simulink model "codeur_qui_marche"  (R2018b)
settings: Solver=VariableStepAuto  StartTime=0.0  StopTime=3  RelTol=1e-3  EnableMultiTasking=on
values from neighbouring files (symbols this model uses):
  freq_proc = 10000    [parametres_cubli.m]
undefined symbols (not defined in the file or in its folder): K3
libraries: c2802xlib x5, c2837xDlib x4, simulink x1, c280xlib x1
settings Model: ExtModeTrigDuration=8  Creator=ntest557  LastModifiedBy=ntest557
settings OptimizationCC: DefaultUnderspecifiedDataType=single  EnhancedBackFolding=on  PassReuseOutputArgsAs=Individual arguments  MaxStackSize=512  OptimizeBlockOrder=speed  DifferentSizesBufferReuse=on  OptimizationCustomize=off
settings DebuggingCC: ParameterTunabilityLossMsg=error
settings HardwareCC: ProdBitPerChar=16  ProdBitPerInt=16  ProdBitPerPointer=32  ProdBitPerSizeT=32  ProdBitPerPtrDiffT=32  ProdLargestAtomicInteger=Integer  ProdLargestAtomicFloat=None  ProdWordSize=16  ProdLongLongMode=on  ProdHWDeviceType=Texas Instruments->C2000
settings SFSimCC: MATLABDynamicMemAlloc=off
settings RTWCC: SystemTargetFile=ert.tlc  HardwareBoard=TI Delfino F28379D LaunchPad  TemplateMakefile=ert_default_tmf  GenerateReport=on  Toolchain=Texas Instruments Code Composer Studio (C2000)  IncludeHyperlinkInReport=on  LaunchReport=on  GenerateTraceInfo=on  GenerateTraceReport=on  GenerateTraceReportSl=on  GenerateTraceReportSf=on  GenerateTraceReportEml=on
settings CodeAppCC: ForceParamTrailComments=on  IgnoreCustomStorageClasses=off  OperatorAnnotations=on  SimulinkDataObjDesc=on  SFDataObjDesc=on  InsertBlockDesc=on
settings ERTTargetCC: CodeReplacementLibrary=TI C28x

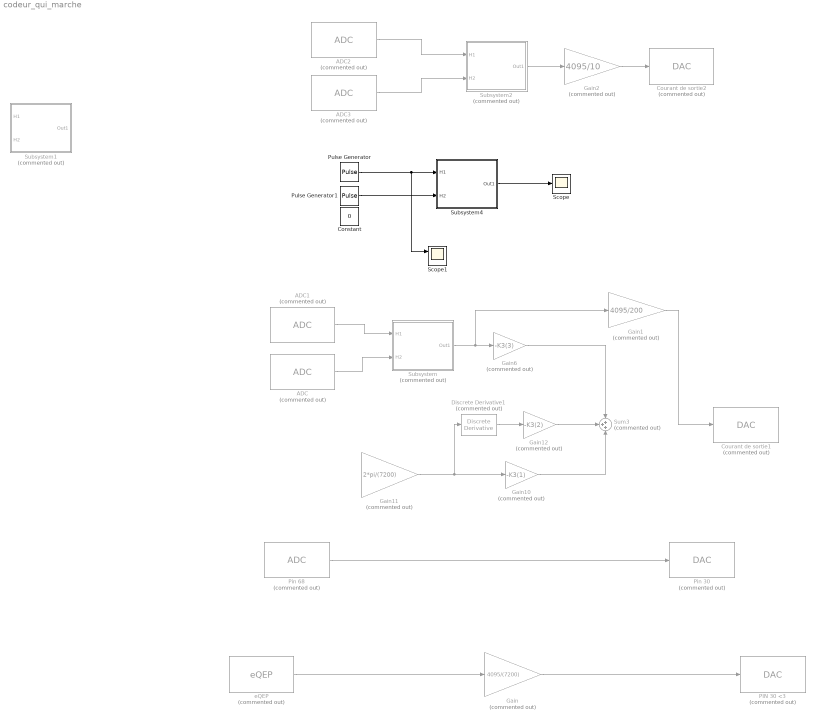
== system codeur_qui_marche ==
  ADC : c2802xlib/ADC  Commented=on  ADCModule=B  samplingMode=Single sample mode  ADCResolution=12-bit (Single-ended input)  useSOC1=SOC0  useSOC2=SOC0_SOC1  SOCAcquisitionWindow=15  SOCTriggerSource=Software  SOCInterruptTrigger=No ADCINT  Ts=1/freq_proc  dType=uint16  postInterrupt=off  interruptSel=ADCINT1  ADCINTContinuous=on  endma=off  chdma=1  blkParamProc=C2000_Type4  conv1=ADCINA0  conv2=ADCINA0 and ADCINB0  conv1_Type4=ADCIN3  conv2_Type4=ADCIN0 and ADCIN1
      settings: SourceProductName=Embedded Coder Support Package for Texas Instruments C2000 Processors
  ADC1 : c2802xlib/ADC  Commented=on  ADCModule=C  samplingMode=Single sample mode  ADCResolution=12-bit (Single-ended input)  useSOC1=SOC0  useSOC2=SOC0_SOC1  SOCAcquisitionWindow=15  SOCTriggerSource=Software  SOCInterruptTrigger=No ADCINT  Ts=1/freq_proc  dType=uint16  postInterrupt=off  interruptSel=ADCINT1  ADCINTContinuous=on  endma=off  chdma=1  blkParamProc=C2000_Type4  conv1=ADCINA0  conv2=ADCINA0 and ADCINB0  conv1_Type4=ADCIN3  conv2_Type4=ADCIN0 and ADCIN1
      settings: SourceProductName=Embedded Coder Support Package for Texas Instruments C2000 Processors
  ADC2 : c2802xlib/ADC  Commented=on  ADCModule=C  samplingMode=Single sample mode  ADCResolution=12-bit (Single-ended input)  useSOC1=SOC0  useSOC2=SOC0_SOC1  SOCAcquisitionWindow=15  SOCTriggerSource=Software  SOCInterruptTrigger=No ADCINT  Ts=1/freq_proc  dType=uint16  postInterrupt=off  interruptSel=ADCINT1  ADCINTContinuous=on  endma=off  chdma=1  blkParamProc=C2000_Type4  conv1=ADCINA0  conv2=ADCINA0 and ADCINB0  conv1_Type4=ADCIN3  conv2_Type4=ADCIN0 and ADCIN1
      settings: SourceProductName=Embedded Coder Support Package for Texas Instruments C2000 Processors
  ADC3 : c2802xlib/ADC  Commented=on  ADCModule=B  samplingMode=Single sample mode  ADCResolution=12-bit (Single-ended input)  useSOC1=SOC0  useSOC2=SOC0_SOC1  SOCAcquisitionWindow=15  SOCTriggerSource=Software  SOCInterruptTrigger=No ADCINT  Ts=1/freq_proc  dType=uint16  postInterrupt=off  interruptSel=ADCINT1  ADCINTContinuous=on  endma=off  chdma=1  blkParamProc=C2000_Type4  conv1=ADCINA0  conv2=ADCINA0 and ADCINB0  conv1_Type4=ADCIN3  conv2_Type4=ADCIN0 and ADCIN1
      settings: SourceProductName=Embedded Coder Support Package for Texas Instruments C2000 Processors
  Constant : Constant  Value=0
  Courant de sortie1 : c2837xDlib/DAC  Commented=on  channel=A  saturate=off
      settings: SourceProductName=Embedded Coder Support Package for Texas Instruments C2000 Processors  SourceProductBaseCode=TIC2000
  Courant de sortie2 : c2837xDlib/DAC  Commented=on  channel=A  saturate=off
      settings: SourceProductName=Embedded Coder Support Package for Texas Instruments C2000 Processors  SourceProductBaseCode=TIC2000
  Discrete Derivative1 : simulink/Discrete/Discrete Derivative  Commented=on  gainval=1.0  ICPrevScaledInput=0.0  OutMin=[]  OutMax=[]  OutDataType=fixdt(1, 16)  OutScaling=2^-10  DoSatur=off
  Gain : Gain  Commented=on  Gain=4095/(7200)
  Gain1 : Gain  Commented=on  Gain=4095/200
  Gain10 : Gain  Commented=on  Gain=-K3(1)
  Gain11 : Gain  Commented=on  Gain=2*pi/(7200)
  Gain12 : Gain  Commented=on  Gain=-K3(2)
  Gain2 : Gain  Commented=on  Gain=4095/10
  Gain6 : Gain  Commented=on  Gain=-K3(3)
  PIN 30 <3 : c2837xDlib/DAC  Commented=on  channel=A  saturate=off
      settings: SourceProductName=Embedded Coder Support Package for Texas Instruments C2000 Processors  SourceProductBaseCode=TIC2000
  Pin 30 : c2837xDlib/DAC  Commented=on  channel=A  saturate=off
      settings: SourceProductName=Embedded Coder Support Package for Texas Instruments C2000 Processors  SourceProductBaseCode=TIC2000
  "Pin 68 " : c2802xlib/ADC  Commented=on  ADCModule=B  samplingMode=Single sample mode  ADCResolution=12-bit (Single-ended input)  useSOC1=SOC0  useSOC2=SOC0_SOC1  SOCAcquisitionWindow=15  SOCTriggerSource=Software  SOCInterruptTrigger=No ADCINT  Ts=0.001  dType=uint16  postInterrupt=off  interruptSel=ADCINT1  ADCINTContinuous=on  endma=off  chdma=1  blkParamProc=C2000_Type4  conv1=ADCINA0  conv2=ADCINA0 and ADCINB0  conv1_Type4=ADCIN4  conv2_Type4=ADCIN0 and ADCIN1
      settings: SourceProductName=Embedded Coder Support Package for Texas Instruments C2000 Processors
  Pulse Generator : DiscretePulseGenerator  PulseType=Time based  Period=0.1  PulseWidth=50
  Pulse Generator1 : DiscretePulseGenerator  PulseType=Time based  Period=0.1  PulseWidth=50  PhaseDelay=2*0.1/3
  Scope : Scope
  Scope1 : Scope  NumInputPorts=2
  Subsystem : Subsystem  Commented=on
  Subsystem1 : Subsystem  Commented=on
  Subsystem2 : Subsystem  Commented=on
  Subsystem4 : Subsystem
  Sum3 : Sum  Commented=on  Inputs=+++
  eQEP : c280xlib/eQEP  Commented=on  useModule=eQEP1  pcInputmode=Quadrature-count  externalClockrate=2x resolution: Count the rising/falling edge  swapPolarityselection=Clockwise  qdfOutputport=off  qapPolarityselection=off  qbpPolarityselection=off  qipPolarityselection=off  qspPolarityselection=off  igatePolarityselection=off  sampleTime=0.0001  pcOutputport=on  pcMaximumvalue=3600*4  indexInitializationcheck=off  indexInitializationevent=Rising edge  strobeInitializationcheck=off  strobeInitializationevent=Rising edge  softwareInitializationcheck=off  softwareInitializationsource=Set to init value at start up  softwareInitializationmode=on  pcInitialvalue=2147483648  pcResetmode=Reset on an index event  ieloutputport=off  indexEventlatch=Rising edge  seloutputport=off  strobeEventlatch=Rising edge  pcefOutputport=off  enableEqepcapture=off  qctmrOutputport=off  qcprdOutputport=off  captureTimerprescaler=128  upEventprescaler=128  overflowErrorflag=off  directionErrorflag=off  captureTimerposition=On position counter read  unitTimerperiod=100000000  captureTimerlatch=off  capturePeriodlatch=off  positionCounterlatch=off  soenPolarityselection=off  spselPolarityselection=Index pin is used for sync output  compareValuesource=Specify via dialog  shadowMode=Load on QPOSCNT=0  compareValue=4294967295  syncOutputwidth=1  polaritySyncoutput=Active high  watchdogEnable=off  watchdogTimer=65535  outport1Datatype=auto  outport2Datatype=auto  outport3Datatype=auto  outport4Datatype=auto  outport5Datatype=auto  outport6Datatype=auto  outport7Datatype=auto  outport8Datatype=auto  outport9Datatype=auto  outport10Datatype=auto  outport11Datatype=auto  outport12Datatype=auto  eqepinterrupt_pce=off  eqepinterrupt_qpe=off  eqepinterrupt_qdc=off  eqepinterrupt_wto=off  eqepinterrupt_pcu=off  eqepinterrupt_pco=off  eqepinterrupt_pcr=off  eqepinterrupt_pcm=off  eqepinterrupt_sel=off  eqepinterrupt_iel=off  eqepinterrupt_uto=off  pheOutputport=off  watchdogOutputport=off  outport13Datatype=auto  outport14Datatype=auto
      settings: SourceProductName=Embedded Coder Support Package for Texas Instruments C2000 Processors  SourceProductBaseCode=TIC2000
  wires:
  "Pin 68 "/1 -> Pin 30/1
  eQEP/1 -> Gain/1
  Gain/1 -> PIN 30 <3/1
  ADC1/1 -> Subsystem/1("H1 ")
  ADC/1 -> Subsystem/2("H2 ")
  Gain12/1 -> Sum3/2
  Gain10/1 -> Sum3/3
  Discrete Derivative1/1 -> Gain12/1
  Subsystem/1(Out1) -> Gain1/1, Gain6/1
  Gain11/1 -> Discrete Derivative1/1, Gain10/1
  Gain6/1 -> Sum3/1
  Gain1/1 -> Courant de sortie1/1
  Subsystem4/1(Out1) -> Scope/1
  Pulse Generator/1 -> Subsystem4/1("H1 "), Scope1/1
  ADC3/1 -> Subsystem2/2("H2 ")
  ADC2/1 -> Subsystem2/1("H1 ")
  Subsystem2/1(Out1) -> Gain2/1
  Gain2/1 -> Courant de sortie2/1
  Pulse Generator1/1 -> Subsystem4/2("H2 ")

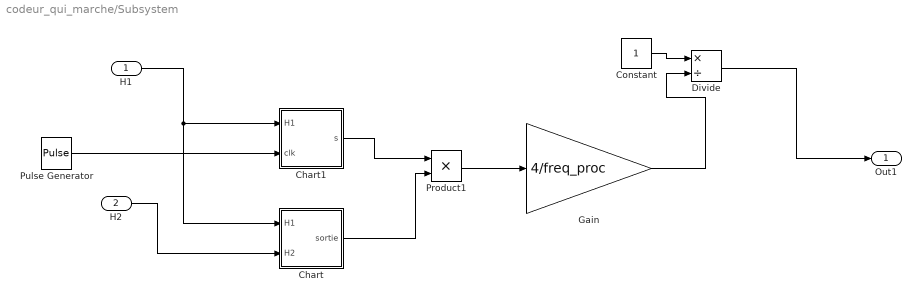
== system codeur_qui_marche/Subsystem ==
  "H1 " : Inport
  "H2 " : Inport  Port=2
  Chart : Stateflow chart  TreatAsAtomicUnit=on
  Chart1 : Stateflow chart  TreatAsAtomicUnit=on
  Constant : Constant
  Divide : Product  Inputs=*/
  Gain : Gain  Gain=4/freq_proc
  Product1 : Product
  Pulse Generator : DiscretePulseGenerator  PulseType=Time based  Period=2/freq_proc  PulseWidth=50
  Out1 : Outport
  wires:
  "H1 "/1 -> Chart/1(H1), Chart1/1(H1)
  Chart/1(sortie) -> Product1/2
  Product1/1 -> Gain/1
  Chart1/1(s) -> Product1/1
  Pulse Generator/1 -> Chart1/2(clk)
  "H2 "/1 -> Chart/2(H2)
  Constant/1 -> Divide/1
  Gain/1 -> Divide/2
  Divide/1 -> Out1/1

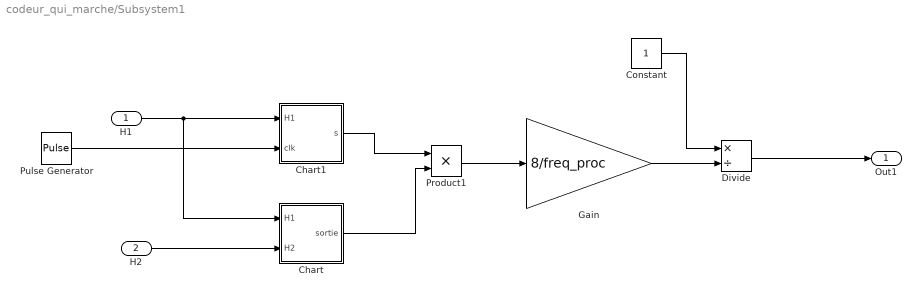
== system codeur_qui_marche/Subsystem1 ==
  "H1 " : Inport
  "H2 " : Inport  Port=2
  Chart : Stateflow chart  TreatAsAtomicUnit=on
  Chart1 : Stateflow chart  TreatAsAtomicUnit=on
  Constant : Constant
  Divide : Product  Inputs=*/
  Gain : Gain  Gain=8/freq_proc
  Product1 : Product
  Pulse Generator : DiscretePulseGenerator  PulseType=Time based  Period=1/freq_proc  PulseWidth=50
  Out1 : Outport
  wires:
  "H1 "/1 -> Chart/1(H1), Chart1/1(H1)
  Chart/1(sortie) -> Product1/2
  Product1/1 -> Gain/1
  Chart1/1(s) -> Product1/1
  Pulse Generator/1 -> Chart1/2(clk)
  "H2 "/1 -> Chart/2(H2)
  Constant/1 -> Divide/1
  Gain/1 -> Divide/2
  Divide/1 -> Out1/1

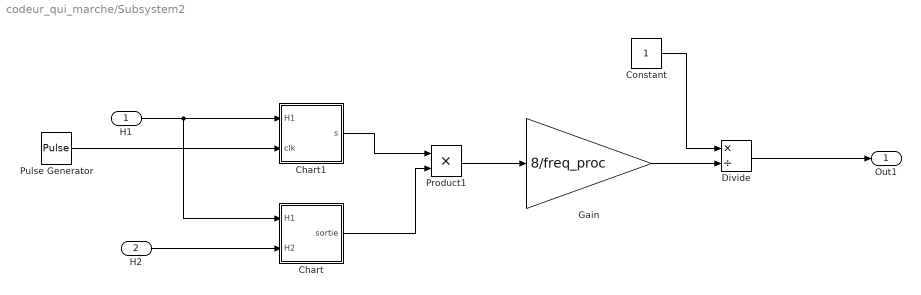
== system codeur_qui_marche/Subsystem2 ==
  "H1 " : Inport
  "H2 " : Inport  Port=2
  Chart : Stateflow chart  TreatAsAtomicUnit=on
  Chart1 : Stateflow chart  TreatAsAtomicUnit=on
  Constant : Constant
  Divide : Product  Inputs=*/
  Gain : Gain  Gain=8/freq_proc
  Product1 : Product
  Pulse Generator : DiscretePulseGenerator  PulseType=Time based  Period=1/freq_proc  PulseWidth=50
  Out1 : Outport
  wires:
  "H1 "/1 -> Chart/1(H1), Chart1/1(H1)
  Chart/1(sortie) -> Product1/2
  Product1/1 -> Gain/1
  Chart1/1(s) -> Product1/1
  Pulse Generator/1 -> Chart1/2(clk)
  "H2 "/1 -> Chart/2(H2)
  Constant/1 -> Divide/1
  Gain/1 -> Divide/2
  Divide/1 -> Out1/1

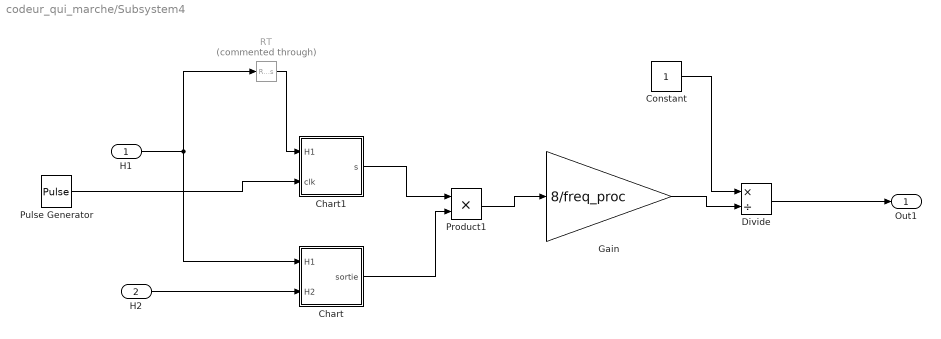
== system codeur_qui_marche/Subsystem4 ==
  "H1 " : Inport
  "H2 " : Inport  Port=2
  Chart : Stateflow chart  TreatAsAtomicUnit=on
  Chart1 : Stateflow chart  TreatAsAtomicUnit=on
  Constant : Constant
  Divide : Product  Inputs=*/
  Gain : Gain  Gain=8/freq_proc
  Product1 : Product
  Pulse Generator : DiscretePulseGenerator  PulseType=Time based  Period=1/freq_proc  PulseWidth=50
  RT : RateTransition  Commented=through  OutPortSampleTime=0.0005
  Out1 : Outport
  wires:
  "H1 "/1 -> Chart/1(H1), RT/1
  Chart/1(sortie) -> Product1/2
  Product1/1 -> Gain/1
  Chart1/1(s) -> Product1/1
  Pulse Generator/1 -> Chart1/2(clk)
  "H2 "/1 -> Chart/2(H2)
  Constant/1 -> Divide/1
  Gain/1 -> Divide/2
  Divide/1 -> Out1/1
  RT/1 -> Chart1/1(H1)

== stateflow chart codeur_qui_marche/Subsystem/Chart ==
  state Test1
  state bas1
    entry: temp = H2;
  state haut1
    entry: temp = H2;
  state bas1descend2
    entry: sortie=1;
  state bas1montant2
    entry: sortie=-1;
  state haut1descend2
    entry: sortie=-1;
  state haut1montant2
    entry: sortie=1;
  state Test2
  state bas2
    entry: temp = H1;
  state haut2
    entry: temp = H1;
  state bas2descend1
    entry: sortie=-1;
  state bas2montant1
    entry: sortie=1;
  state haut2descend1
    entry: sortie=1;
  state haut2montant1
    entry: sortie=-1;
  (default) -> Test1
  bas2montant1 -> Test1
  haut2descend1 -> Test1
  bas2descend1 -> Test1
  haut2montant1 -> Test1
  Test1 -> bas1 [order 2] : [H1<=0]
  Test1 -> haut1 [order 1] : [H1>0]
  haut1 -> haut1montant2 [order 1] : [H2>temp]
  haut1 -> haut1descend2 [order 2] : [H2<temp]
  bas1 -> bas1descend2 [order 2] : [H2<temp]
  bas1 -> bas1montant2 [order 1] : [H2>temp]
  bas1descend2 -> Test2
  bas1montant2 -> Test2
  haut1descend2 -> Test2
  haut1montant2 -> Test2
  Test2 -> haut2 [order 1] : [H2>0]
  Test2 -> bas2 [order 2] : [H2<=0]
  haut2 -> haut2descend1 [order 2] : [H1<temp]
  haut2 -> haut2montant1 [order 1] : [H1>temp]
  bas2 -> bas2descend1 [order 2] : [H1<temp]
  bas2 -> bas2montant1 [order 1] : [H1>temp]
  data: H1 input; H2 input; sortie output; temp local

== stateflow chart codeur_qui_marche/Subsystem1/Chart ==
  state Test1
  state bas1
    entry: temp = H2;
  state haut1
    entry: temp = H2;
  state bas1descend2
    entry: sortie=1;
  state bas1montant2
    entry: sortie=-1;
  state haut1descend2
    entry: sortie=-1;
  state haut1montant2
    entry: sortie=1;
  state Test2
  state bas2
    entry: temp = H1;
  state haut2
    entry: temp = H1;
  state bas2descend1
    entry: sortie=-1;
  state bas2montant1
    entry: sortie=1;
  state haut2descend1
    entry: sortie=1;
  state haut2montant1
    entry: sortie=-1;
  (default) -> Test1
  bas2montant1 -> Test1
  haut2descend1 -> Test1
  bas2descend1 -> Test1
  haut2montant1 -> Test1
  Test1 -> bas1 [order 2] : [H1<=0.5]
  Test1 -> haut1 [order 1] : [H1>0.5]
  haut1 -> haut1montant2 [order 1] : [H2>temp]
  haut1 -> haut1descend2 [order 2] : [H2<temp]
  bas1 -> bas1descend2 [order 2] : [H2<temp]
  bas1 -> bas1montant2 [order 1] : [H2>temp]
  bas1descend2 -> Test2
  bas1montant2 -> Test2
  haut1descend2 -> Test2
  haut1montant2 -> Test2
  Test2 -> haut2 [order 1] : [H2>0.5]
  Test2 -> bas2 [order 2] : [H2<=0.5]
  haut2 -> haut2descend1 [order 2] : [H1<temp]
  haut2 -> haut2montant1 [order 1] : [H1>temp]
  bas2 -> bas2descend1 [order 2] : [H1<temp]
  bas2 -> bas2montant1 [order 1] : [H1>temp]
  data: H1 input; H2 input; sortie output; temp local

== stateflow chart codeur_qui_marche/Subsystem/Chart1 ==
  state bot1
    entry: s = 0;
    entry: compteur=-1;
  state top
    entry: compteur=compteur+1;
  state top2
  state wait
  state top3
    entry: compteur=compteur+1;
  state top4
  state top1
    entry: s=compteur;
    compteur=-1;
  state wait1
  state top5
    entry: s=compteur;
    compteur=-1;
  (default) -> bot1
  bot1 -> top : [H1>0.5]
  top2 -> top : [clk==1]
  wait -> top2 : [clk==0]
  top5 -> top : [clk==1]
  top -> top1 [order 1] : [H1<=0.5]
  top -> wait [order 2] : [H1>0.5]
  top4 -> top3 : [clk==1]
  top1 -> top3 : [clk==1]
  top3 -> top5 [order 1] : [H1>0.5]
  top3 -> wait1 [order 2] : [H1<=0.5]
  wait1 -> top4 : [clk==0]
  data: s output; H1 input; clk input; compteur local

== stateflow chart codeur_qui_marche/Subsystem1/Chart1 ==
  state bot1
    entry: s = 0;
    entry: compteur=-1;
  state top
    entry: compteur=compteur+1;
  state top2
  state wait
  state top3
    entry: compteur=compteur+1;
  state top4
  state top1
    entry: s=compteur;
    compteur=-1;
  state wait1
  state top5
    entry: s=compteur;
    compteur=-1;
  (default) -> bot1
  bot1 -> top : [H1>0.5]
  top2 -> top : [clk==1]
  wait -> top2 : [clk==0]
  top5 -> top : [clk==1]
  top -> top1 [order 1] : [H1<=0.5]
  top -> wait [order 2] : [H1>0.5]
  top4 -> top3 : [clk==1]
  top1 -> top3 : [clk==1]
  top3 -> top5 [order 1] : [H1>0.5]
  top3 -> wait1 [order 2] : [H1<=0.5]
  wait1 -> top4 : [clk==0]
  data: s output; H1 input; clk input; compteur local

== stateflow chart codeur_qui_marche/Subsystem2/Chart ==
  state Test1
  state bas1
    entry: temp = H2;
  state haut1
    entry: temp = H2;
  state bas1descend2
    entry: sortie=1;
  state bas1montant2
    entry: sortie=-1;
  state haut1descend2
    entry: sortie=-1;
  state haut1montant2
    entry: sortie=1;
  state Test2
  state bas2
    entry: temp = H1;
  state haut2
    entry: temp = H1;
  state bas2descend1
    entry: sortie=-1;
  state bas2montant1
    entry: sortie=1;
  state haut2descend1
    entry: sortie=1;
  state haut2montant1
    entry: sortie=-1;
  (default) -> Test1
  bas2montant1 -> Test1
  haut2descend1 -> Test1
  bas2descend1 -> Test1
  haut2montant1 -> Test1
  Test1 -> bas1 [order 2] : [H1<=0.5]
  Test1 -> haut1 [order 1] : [H1>0.5]
  haut1 -> haut1montant2 [order 1] : [H2>temp]
  haut1 -> haut1descend2 [order 2] : [H2<temp]
  bas1 -> bas1descend2 [order 2] : [H2<temp]
  bas1 -> bas1montant2 [order 1] : [H2>temp]
  bas1descend2 -> Test2
  bas1montant2 -> Test2
  haut1descend2 -> Test2
  haut1montant2 -> Test2
  Test2 -> haut2 [order 1] : [H2>0.5]
  Test2 -> bas2 [order 2] : [H2<=0.5]
  haut2 -> haut2descend1 [order 2] : [H1<temp]
  haut2 -> haut2montant1 [order 1] : [H1>temp]
  bas2 -> bas2descend1 [order 2] : [H1<temp]
  bas2 -> bas2montant1 [order 1] : [H1>temp]
  data: H1 input; H2 input; sortie output; temp local

== stateflow chart codeur_qui_marche/Subsystem2/Chart1 ==
  state bot1
    entry: s = 0;
    entry: compteur=-1;
  state top
    entry: compteur=compteur+1;
  state top2
  state wait
  state top3
    entry: compteur=compteur+1;
  state top4
  state top1
    entry: s=compteur;
    compteur=-1;
  state wait1
  state top5
    entry: s=compteur;
    compteur=-1;
  (default) -> bot1
  bot1 -> top : [H1>0.5]
  top2 -> top : [clk==1]
  wait -> top2 : [clk==0]
  top5 -> top : [clk==1]
  top -> top1 [order 1] : [H1<=0.5]
  top -> wait [order 2] : [H1>0.5]
  top4 -> top3 : [clk==1]
  top1 -> top3 : [clk==1]
  top3 -> top5 [order 1] : [H1>0.5]
  top3 -> wait1 [order 2] : [H1<=0.5]
  wait1 -> top4 : [clk==0]
  data: s output; H1 input; clk input; compteur local

== stateflow chart codeur_qui_marche/Subsystem4/Chart ==
  state Test3
    entry: sortie=1000;
  state Test1
  state bas1
    entry: temp = H2;
  state haut1
    entry: temp = H2;
  state bas1descend2
    entry: sortie=1;
  state bas1montant2
    entry: sortie=-1;
  state haut1descend2
    entry: sortie=-1;
  state haut1montant2
    entry: sortie=1;
  state Test2
  state bas2
    entry: temp = H1;
  state haut2
    entry: temp = H1;
  state bas2descend1
    entry: sortie=-1;
  state bas2montant1
    entry: sortie=1;
  state haut2descend1
    entry: sortie=1;
  state haut2montant1
    entry: sortie=-1;
  (default) -> Test3
  Test3 -> Test1
  bas2montant1 -> Test1
  haut2descend1 -> Test1
  bas2descend1 -> Test1
  haut2montant1 -> Test1
  Test1 -> bas1 [order 2] : [H1<=0.5]
  Test1 -> haut1 [order 1] : [H1>0.5]
  haut1 -> haut1montant2 [order 1] : [H2>temp+0.2]
  haut1 -> haut1descend2 [order 2] : [H2<temp-0.2]
  bas1 -> bas1descend2 [order 2] : [H2<temp-0.2]
  bas1 -> bas1montant2 [order 1] : [H2>temp+0.2]
  bas1descend2 -> Test2
  bas1montant2 -> Test2
  haut1descend2 -> Test2
  haut1montant2 -> Test2
  Test2 -> haut2 [order 1] : [H2>0.5]
  Test2 -> bas2 [order 2] : [H2<=0.5]
  haut2 -> haut2descend1 [order 2] : [H1<temp-0.2]
  haut2 -> haut2montant1 [order 1] : [H1>temp+0.2]
  bas2 -> bas2descend1 [order 2] : [H1<temp-0.2]
  bas2 -> bas2montant1 [order 1] : [H1>temp+0.2]
  data: H1 input; H2 input; sortie output; temp local

== stateflow chart codeur_qui_marche/Subsystem4/Chart1 ==
  state bot1
    entry: s = 0;
    entry: compteur=-1;
  state top
    entry: compteur=compteur+1;
  state top2
  state wait
  state top3
    entry: compteur=compteur+1;
  state top4
  state top1
    entry: s=compteur;
    compteur=-1;
  state wait1
  state top5
    entry: s=compteur;
    compteur=-1;
  (default) -> bot1
  bot1 -> top : [H1>0.5]
  top2 -> top : [clk==1]
  wait -> top2 : [clk==0]
  top5 -> top : [clk==1]
  top -> top1 [order 1] : [H1<=0.5]
  top -> wait [order 2] : [H1>0.5]
  top4 -> top3 : [clk==1]
  top1 -> top3 : [clk==1]
  top3 -> top5 [order 1] : [H1>0.5]
  top3 -> wait1 [order 2] : [H1<=0.5]
  wait1 -> top4 : [clk==0]
  data: s output; H1 input; clk input; compteur local
